simulink model "NLD1"  (R2022a)
settings: Solver=FixedStepDiscrete  StartTime=0.0  StopTime=xin.TimeInfo.End  RelTol=1e-3
values from neighbouring files (symbols this model uses):
  Ts = 1e-6    (= 1e-06)    [NLD1sim.m]    (also in NLD2sim.m; SPNF1sim.m; SPNF2sim.m)
undefined symbols (not defined in the file or in its folder): cols
settings Model: Creator=dileepan  LastModifiedBy=dileepan
settings SolverCC: AlgebraicLoopSolver=TrustRegion
settings DataIOCC: SaveFormat=Array  SaveOutput=off  SignalLogging=off  DSMLogging=off  SaveTime=off  ReturnWorkspaceOutputs=off
settings DebuggingCC: UnconnectedInputMsg=warning  UnconnectedOutputMsg=warning  UnconnectedLineMsg=warning  SFMachineParentedDataDiag=warning
settings RTWCC: DLArmComputeVersion=19.05

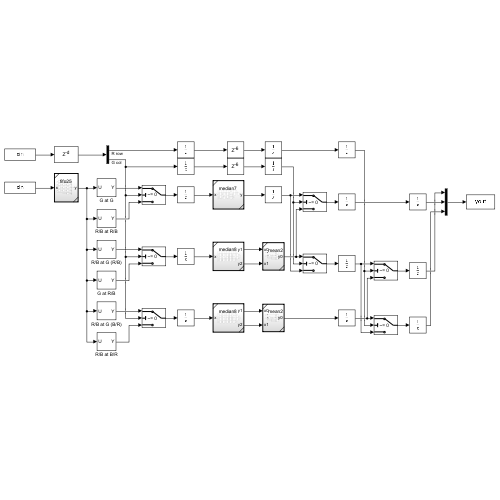
[thumbnail: Simulink's stored preview of the top-level diagram]
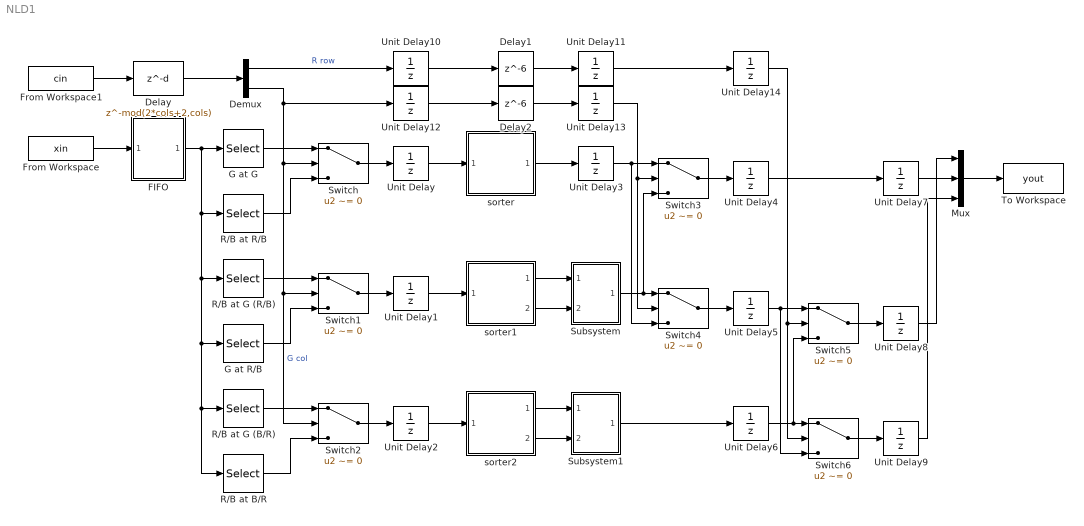
== system NLD1 ==
  Delay : Delay  DelayLength=mod(2*cols+2,cols)
  Delay1 : Delay  DelayLength=6
  Delay2 : Delay  DelayLength=6
  Demux : Demux  Outputs=2
  FIFO : Subsystem  TreatAsAtomicUnit=on  ReferencedSubsystem=fifo25
  From Workspace : FromWorkspace  VariableName=xin  SampleTime=Ts
  From Workspace1 : FromWorkspace  VariableName=cin  SampleTime=Ts
  G at G : Selector  InputPortWidth=25  IndexOptions=Index vector (dialog)  Indices=[7 9 13 13 13 17 19]  OutputSizes=1
  G at R/B : Selector  InputPortWidth=25  IndexOptions=Index vector (dialog)  Indices=[8 8 12 12 14 14 18 18]  OutputSizes=1
  Mux : Mux  Inputs=3
  R/B at B/R : Selector  InputPortWidth=25  IndexOptions=Index vector (dialog)  Indices=[7 7 9 9 17 17 19 19]  OutputSizes=1
  R/B at G (B/R) : Selector  InputPortWidth=25  IndexOptions=Index vector (dialog)  Indices=[6 8 8 10 16 18 18 20]  OutputSizes=1
  R/B at G (R/B) : Selector  InputPortWidth=25  IndexOptions=Index vector (dialog)  Indices=[2 4 12 12 14 14 22 24]  OutputSizes=1
  R/B at R/B : Selector  InputPortWidth=25  IndexOptions=Index vector (dialog)  Indices=[3 11 13 13 13 15 23]  OutputSizes=1
  Subsystem : Subsystem  TreatAsAtomicUnit=on  ReferencedSubsystem=mean2
  Subsystem1 : Subsystem  TreatAsAtomicUnit=on  ReferencedSubsystem=mean2
  Switch{,1..6} (7 alike) : Switch  Criteria=u2 ~= 0  SaturateOnIntegerOverflow=off  InputSameDT=off
  To Workspace : ToWorkspace  VariableName=yout  SaveFormat=Timeseries  SampleTime=-1
  Unit Delay{,1..14} (15 alike) : UnitDelay  SampleTime=-1  HasFrameUpgradeWarning=on
  sorter : Subsystem  TreatAsAtomicUnit=on  ReferencedSubsystem=median7
  sorter1 : Subsystem  TreatAsAtomicUnit=on  ReferencedSubsystem=median8
  sorter2 : Subsystem  TreatAsAtomicUnit=on  ReferencedSubsystem=median8
  wires:
  From Workspace1/1 -> Delay/1
  G at G/1 -> Switch/1
  R/B at R/B/1 -> Switch/3
  From Workspace/1 -> FIFO/1
  R/B at G (R/B)/1 -> Switch1/1
  G at R/B/1 -> Switch1/3
  R/B at B/R/1 -> Switch2/3
  R/B at G (B/R)/1 -> Switch2/1
  Mux/1 -> To Workspace/1
  Demux/2 -> Switch/2, Switch1/2, Switch2/2, Unit Delay12/1  "G col"
  FIFO/1 -> G at G/1, R/B at R/B/1, R/B at G (R/B)/1, G at R/B/1, R/B at G (B/R)/1, R/B at B/R/1
  Switch/1 -> Unit Delay/1
  Switch1/1 -> Unit Delay1/1
  Switch2/1 -> Unit Delay2/1
  Unit Delay/1 -> sorter/1
  Unit Delay1/1 -> sorter1/1
  Unit Delay2/1 -> sorter2/1
  sorter/1 -> Unit Delay3/1
  sorter1/1 -> Subsystem/1
  sorter1/2 -> Subsystem/2
  sorter2/2 -> Subsystem1/2
  sorter2/1 -> Subsystem1/1
  Delay/1 -> Demux/1
  Subsystem/1 -> Switch3/3, Switch4/1
  Unit Delay3/1 -> Switch4/3, Switch3/1
  Switch3/1 -> Unit Delay4/1
  Switch4/1 -> Unit Delay5/1
  Subsystem1/1 -> Unit Delay6/1
  Unit Delay5/1 -> Switch6/3, Switch5/1
  Unit Delay6/1 -> Switch5/3, Switch6/1
  Switch5/1 -> Unit Delay8/1
  Switch6/1 -> Unit Delay9/1
  Unit Delay4/1 -> Unit Delay7/1
  Unit Delay7/1 -> Mux/2
  Unit Delay8/1 -> Mux/1
  Unit Delay9/1 -> Mux/3
  Demux/1 -> Unit Delay10/1  "R row"
  Unit Delay10/1 -> Delay1/1
  Delay1/1 -> Unit Delay11/1
  Unit Delay12/1 -> Delay2/1
  Delay2/1 -> Unit Delay13/1
  Unit Delay13/1 -> Switch3/2, Switch4/2
  Unit Delay11/1 -> Unit Delay14/1
  Unit Delay14/1 -> Switch5/2, Switch6/2
